simulink model "fft_wideband_real"  (R2012b)
settings: Solver=ode45  StartTime=0.0  StopTime=19999  RelTol=1e-3
undefined symbols (not defined in the file): fft_wideband_real_shift_schedule_user_data_out
libraries: xbsIndex_r4 x8703, xbsReplacements_r4 x36, xps_library x24, dspsigops x16, simulink_xsg_bridge x1
(part 1 of 51)
settings Model: Creator=sgowda  LastModifiedBy=sgowda

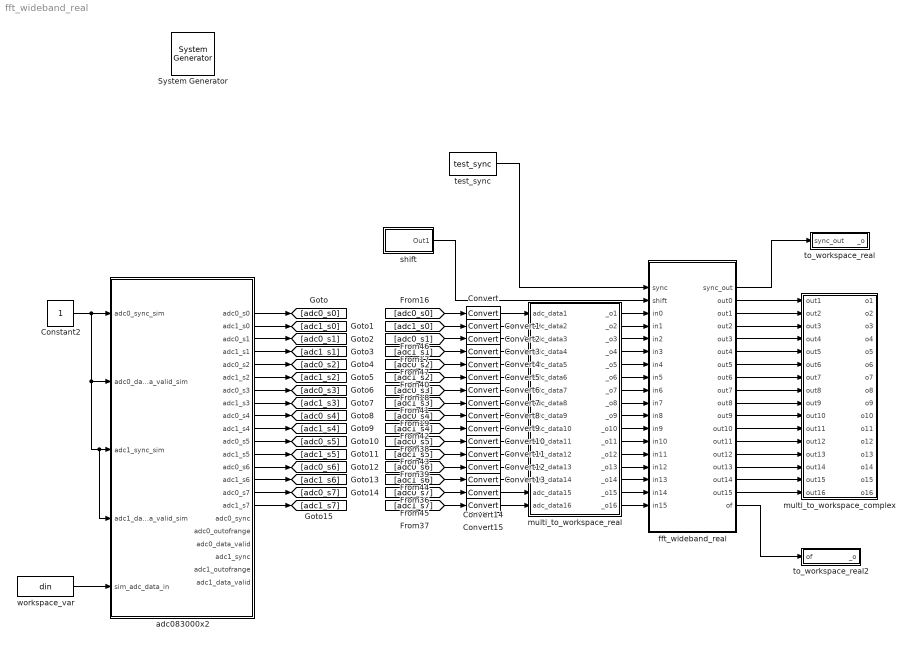
== system fft_wideband_real ==
  " System Generator" : xbsIndex_r4/ System Generator  Tag=genX  xilinxfamily=Kintex7  part=xc7k325t  speed=-3  package=fbg676  synthesis_tool=XST  clock_wrapper=Clock Enables  directory=./netlist  proj_type=Project Navigator  Synth_file=XST Defaults  Impl_file=ISE Defaults  testbench=off  simulink_period=1  sysclk_period=10  dcm_input_clock_period=10  incr_netlist=off  trim_vbits=Everywhere in SubSystem  dbl_ovrd=According to Block Masks  core_generation=According to Block Masks  run_coregen=off  deprecated_control=off  eval_field=0  block_type=sysgen
  Constant2 : Constant
  Convert{,1..15} (16 alike) : xbsIndex_r4/Convert  gui_display_data_type=Fixed-point  arith_type="Signed  (2's comp)"  n_bits=18  bin_pt=17  float_type=Single  exp_bits=8  fraction_bits=24  quantization=Truncate  overflow=Wrap  en=off  latency=0  dbl_ovrd=off  pipeline=off  block_type=convert
  adc083000x2 : Subsystem  Tag=xps:adc083000x2  mask(adc_083000x2){use_adc0=on, use_adc1=on, demux_adc=off, clock_sync=on, verbose=off, using_ctrl=off, adc_clk_rate=1500, sample_period=1, bit_width=8}
      mask prompts: use_adc0 "Use ZD0K0?"; use_adc1 "Use ZDOK1?"; demux_adc "Demux ADCs by 2?"; clock_sync "Interleave 2 ADC boards?"; verbose "Verbose Block Creation?"; using_ctrl "Add ports for control registers?"; adc_clk_rate "ADC clock rate (MHz)"; sample_period "Sample Period"; bit_width "Output Bit Width"
      mask help:
      | The ADC block converts analog inputs to digital outputs.
      | Every clock cycle, the inputs are sampled and digitized to
      | 8 bit binary point numbers in the range of [-1, 1).
      |
      | Online block-specific documentation: http://casper.berkeley.edu/wiki/Adc083000
      mask init:
      | adc083000_mask;
      mask Help: eval('xlWeb([getenv(''MLIB_ROOT''), ''\doc\html\sys_adc\sys_adc.html''])')
  fft_wideband_real : Subsystem
  multi_to_workspace_complex : Subsystem  mask{var_name=out, n_bits=18, bin_pt=17, n_inputs=16}
      mask prompts: var_name "Workspace variable name"; n_bits "# of bits"; bin_pt "Binary Point"; n_inputs "# of inputs"
      mask init:
      | config.source = str2func('multi_mat_output_data_cplx_init_xblock');
      | config.toplevel = gcb();
      | xBlock(config, {config.toplevel, 'var_name', var_name, ...
      |     'n_bits', n_bits, 'bin_pt', bin_pt, 'n_inputs', n_inputs});
  multi_to_workspace_real : Subsystem  mask{var_name=adc_data, n_inputs=16}
      mask prompts: var_name "Workspace variable name"; n_inputs "# of inputs"
      mask init:
      | config.source = str2func('multi_mat_output_data_init_xblock');
      | config.toplevel = gcb();
      | xBlock(config, {config.toplevel, 'var_name', var_name, 'n_inputs', n_inputs});
  shift : Subsystem  mask{shift_schedule=0}
      mask prompts: shift_schedule "Shift schedule"
  test_sync : simulink_xsg_bridge/test_sync
  to_workspace_real : Subsystem  mask{var_name=sync_out}
      mask prompts: var_name "Workspace variable name"
      mask init:
      | config.source = str2func('mat_output_data_init_xblock');
      | config.toplevel = gcb();
      | xBlock(config, {config.toplevel, 'var_name', var_name});
  to_workspace_real2 : Subsystem  mask{var_name=of}
      mask prompts: var_name "Workspace variable name"
      mask init:
      | config.source = str2func('mat_output_data_init_xblock');
      | config.toplevel = gcb();
      | xBlock(config, {config.toplevel, 'var_name', var_name});
  workspace_var : FromWorkspace  VariableName=din
  wires:
  adc083000x2/1(adc0_s0) -> [adc0_s0]
  adc083000x2/2(adc1_s0) -> [adc1_s0]
  adc083000x2/3(adc0_s1) -> [adc0_s1]
  adc083000x2/4(adc1_s1) -> [adc1_s1]
  adc083000x2/5(adc0_s2) -> [adc0_s2]
  adc083000x2/6(adc1_s2) -> [adc1_s2]
  adc083000x2/7(adc0_s3) -> [adc0_s3]
  adc083000x2/8(adc1_s3) -> [adc1_s3]
  adc083000x2/9(adc0_s4) -> [adc0_s4]
  adc083000x2/10(adc1_s4) -> [adc1_s4]
  adc083000x2/11(adc0_s5) -> [adc0_s5]
  adc083000x2/12(adc1_s5) -> [adc1_s5]
  adc083000x2/13(adc0_s6) -> [adc0_s6]
  adc083000x2/14(adc1_s6) -> [adc1_s6]
  adc083000x2/15(adc0_s7) -> [adc0_s7]
  adc083000x2/16(adc1_s7) -> [adc1_s7]
  Constant2/1 -> adc083000x2/2(adc0_data_valid_sim), adc083000x2/3(adc1_sync_sim), adc083000x2/4(adc1_data_valid_sim), adc083000x2/1(adc0_sync_sim)
  workspace_var/1 -> adc083000x2/5(sim_adc_data_in)
  [adc0_s0] -> Convert/1
  [adc1_s0] -> Convert1/1
  [adc0_s1] -> Convert2/1
  [adc1_s1] -> Convert3/1
  [adc0_s2] -> Convert4/1
  [adc1_s2] -> Convert5/1
  [adc0_s3] -> Convert6/1
  [adc1_s3] -> Convert7/1
  [adc0_s4] -> Convert8/1
  [adc1_s4] -> Convert9/1
  [adc0_s5] -> Convert10/1
  [adc1_s5] -> Convert11/1
  [adc0_s6] -> Convert12/1
  [adc1_s6] -> Convert13/1
  [adc0_s7] -> Convert14/1
  [adc1_s7] -> Convert15/1
  test_sync/1 -> fft_wideband_real/1(sync)
  fft_wideband_real/1(sync_out) -> to_workspace_real/1(sync_out)
  shift/1(Out1) -> fft_wideband_real/2(shift)
  fft_wideband_real/2(out0) -> multi_to_workspace_complex/1(out1)
  fft_wideband_real/3(out1) -> multi_to_workspace_complex/2(out2)
  fft_wideband_real/4(out2) -> multi_to_workspace_complex/3(out3)
  fft_wideband_real/5(out3) -> multi_to_workspace_complex/4(out4)
  fft_wideband_real/6(out4) -> multi_to_workspace_complex/5(out5)
  fft_wideband_real/7(out5) -> multi_to_workspace_complex/6(out6)
  fft_wideband_real/8(out6) -> multi_to_workspace_complex/7(out7)
  fft_wideband_real/9(out7) -> multi_to_workspace_complex/8(out8)
  fft_wideband_real/10(out8) -> multi_to_workspace_complex/9(out9)
  fft_wideband_real/11(out9) -> multi_to_workspace_complex/10(out10)
  fft_wideband_real/12(out10) -> multi_to_workspace_complex/11(out11)
  fft_wideband_real/13(out11) -> multi_to_workspace_complex/12(out12)
  fft_wideband_real/14(out12) -> multi_to_workspace_complex/13(out13)
  fft_wideband_real/15(out13) -> multi_to_workspace_complex/14(out14)
  fft_wideband_real/16(out14) -> multi_to_workspace_complex/15(out15)
  fft_wideband_real/17(out15) -> multi_to_workspace_complex/16(out16)
  fft_wideband_real/18(of) -> to_workspace_real2/1(of)
  Convert3/1 -> multi_to_workspace_real/4(adc_data4)
  Convert9/1 -> multi_to_workspace_real/10(adc_data10)
  Convert13/1 -> multi_to_workspace_real/14(adc_data14)
  Convert14/1 -> multi_to_workspace_real/15(adc_data15)
  Convert15/1 -> multi_to_workspace_real/16(adc_data16)
  Convert5/1 -> multi_to_workspace_real/6(adc_data6)
  Convert1/1 -> multi_to_workspace_real/2(adc_data2)
  Convert11/1 -> multi_to_workspace_real/12(adc_data12)
  Convert/1 -> multi_to_workspace_real/1(adc_data1)
  Convert10/1 -> multi_to_workspace_real/11(adc_data11)
  Convert12/1 -> multi_to_workspace_real/13(adc_data13)
  Convert2/1 -> multi_to_workspace_real/3(adc_data3)
  Convert4/1 -> multi_to_workspace_real/5(adc_data5)
  Convert6/1 -> multi_to_workspace_real/7(adc_data7)
  Convert7/1 -> multi_to_workspace_real/8(adc_data8)
  Convert8/1 -> multi_to_workspace_real/9(adc_data9)
  multi_to_workspace_real/13(_o13) -> fft_wideband_real/15(in12)
  multi_to_workspace_real/11(_o11) -> fft_wideband_real/13(in10)
  multi_to_workspace_real/3(_o3) -> fft_wideband_real/5(in2)
  multi_to_workspace_real/1(_o1) -> fft_wideband_real/3(in0)
  multi_to_workspace_real/4(_o4) -> fft_wideband_real/6(in3)
  multi_to_workspace_real/5(_o5) -> fft_wideband_real/7(in4)
  multi_to_workspace_real/8(_o8) -> fft_wideband_real/10(in7)
  multi_to_workspace_real/7(_o7) -> fft_wideband_real/9(in6)
  multi_to_workspace_real/14(_o14) -> fft_wideband_real/16(in13)
  multi_to_workspace_real/12(_o12) -> fft_wideband_real/14(in11)
  multi_to_workspace_real/16(_o16) -> fft_wideband_real/18(in15)
  multi_to_workspace_real/15(_o15) -> fft_wideband_real/17(in14)
  multi_to_workspace_real/6(_o6) -> fft_wideband_real/8(in5)
  multi_to_workspace_real/9(_o9) -> fft_wideband_real/11(in8)
  multi_to_workspace_real/2(_o2) -> fft_wideband_real/4(in1)
  multi_to_workspace_real/10(_o10) -> fft_wideband_real/12(in9)

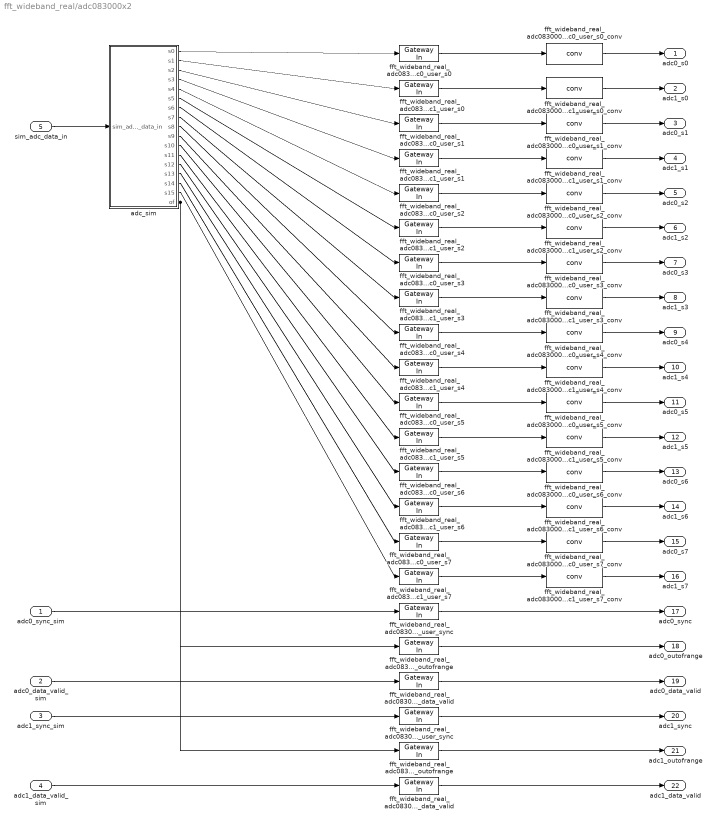
== system fft_wideband_real/adc083000x2 ==
  adc0_sync_sim : Inport
  adc0_data_valid_sim : Inport  Port=2
  adc1_sync_sim : Inport  Port=3
  adc1_data_valid_sim : Inport  Port=4
  sim_adc_data_in : Inport  Port=5
  adc_sim : Subsystem  AncestorBlock=xps_library/ADCs/adc_sim  mask(adc_sim){nStreams=16, bit_width=8}
      mask prompts: nStreams "Number of Output Streams"; bit_width "Sample Bit Width"
      mask help:
      | This block simulates the behavior of a demuxed ADC, which takes
      | as input a waveform and returns digital samples in parallel at
      | a slower rate.
      |
      | This block is used to simulate the behavior
      mask init:
      | adc_sim_init(gcb, ...
      |     'nStreams', nStreams, ...
      |     'bit_width', bit_width);
  fft_wideband_real_adc083000x2_adc0_user_data_valid : xbsIndex_r4/Gateway In  gui_display_data_type=Fixed-point  arith_type=Unsigned  n_bits=1  bin_pt=0  preci_type=Single  exp_width=8  frac_width=24  quantization="Round  (unbiased: +/- Inf)"  overflow=Saturate  period=1  dbl_ovrd=off  timing_constraint=None  locs_specified=off  LOCs={}  UseAsADC=off  ADCChannel='1'  inherit_from_input=off  hdl_port=on  block_type=gatewayin
  fft_wideband_real_adc083000x2_adc0_user_outofrange : xbsIndex_r4/Gateway In  gui_display_data_type=Fixed-point  arith_type=Unsigned  n_bits=4  bin_pt=0  preci_type=Single  exp_width=8  frac_width=24  quantization="Round  (unbiased: +/- Inf)"  overflow=Saturate  period=1  dbl_ovrd=off  timing_constraint=None  locs_specified=off  LOCs={}  UseAsADC=off  ADCChannel='1'  inherit_from_input=off  hdl_port=on  block_type=gatewayin
  fft_wideband_real_adc083000x2_adc0_user_s{0..7} (8 alike) : xbsIndex_r4/Gateway In  gui_display_data_type=Fixed-point  arith_type=Unsigned  n_bits=8  bin_pt=0  preci_type=Single  exp_width=8  frac_width=24  quantization="Round  (unbiased: +/- Inf)"  overflow=Saturate  period=1  dbl_ovrd=off  timing_constraint=None  locs_specified=off  LOCs={}  UseAsADC=off  ADCChannel='1'  inherit_from_input=off  hdl_port=on  block_type=gatewayin
  fft_wideband_real_adc083000x2_adc0_user_s0_conv : xps_library/ADCs/conv  bit_width=8
  fft_wideband_real_adc083000x2_adc0_user_s1_conv : xps_library/ADCs/conv  bit_width=8
  fft_wideband_real_adc083000x2_adc0_user_s2_conv : xps_library/ADCs/conv  bit_width=8
  fft_wideband_real_adc083000x2_adc0_user_s3_conv : xps_library/ADCs/conv  bit_width=8
  fft_wideband_real_adc083000x2_adc0_user_s4_conv : xps_library/ADCs/conv  bit_width=8
  fft_wideband_real_adc083000x2_adc0_user_s5_conv : xps_library/ADCs/conv  bit_width=8
  fft_wideband_real_adc083000x2_adc0_user_s6_conv : xps_library/ADCs/conv  bit_width=8
  fft_wideband_real_adc083000x2_adc0_user_s7_conv : xps_library/ADCs/conv  bit_width=8
  fft_wideband_real_adc083000x2_adc0_user_sync : xbsIndex_r4/Gateway In  gui_display_data_type=Fixed-point  arith_type=Unsigned  n_bits=4  bin_pt=0  preci_type=Single  exp_width=8  frac_width=24  quantization="Round  (unbiased: +/- Inf)"  overflow=Saturate  period=1  dbl_ovrd=off  timing_constraint=None  locs_specified=off  LOCs={}  UseAsADC=off  ADCChannel='1'  inherit_from_input=off  hdl_port=on  block_type=gatewayin
  fft_wideband_real_adc083000x2_adc1_user_data_valid : xbsIndex_r4/Gateway In  gui_display_data_type=Fixed-point  arith_type=Unsigned  n_bits=1  bin_pt=0  preci_type=Single  exp_width=8  frac_width=24  quantization="Round  (unbiased: +/- Inf)"  overflow=Saturate  period=1  dbl_ovrd=off  timing_constraint=None  locs_specified=off  LOCs={}  UseAsADC=off  ADCChannel='1'  inherit_from_input=off  hdl_port=on  block_type=gatewayin
  fft_wideband_real_adc083000x2_adc1_user_outofrange : xbsIndex_r4/Gateway In  gui_display_data_type=Fixed-point  arith_type=Unsigned  n_bits=4  bin_pt=0  preci_type=Single  exp_width=8  frac_width=24  quantization="Round  (unbiased: +/- Inf)"  overflow=Saturate  period=1  dbl_ovrd=off  timing_constraint=None  locs_specified=off  LOCs={}  UseAsADC=off  ADCChannel='1'  inherit_from_input=off  hdl_port=on  block_type=gatewayin
  fft_wideband_real_adc083000x2_adc1_user_s{0..7} (8 alike) : xbsIndex_r4/Gateway In  gui_display_data_type=Fixed-point  arith_type=Unsigned  n_bits=8  bin_pt=0  preci_type=Single  exp_width=8  frac_width=24  quantization="Round  (unbiased: +/- Inf)"  overflow=Saturate  period=1  dbl_ovrd=off  timing_constraint=None  locs_specified=off  LOCs={}  UseAsADC=off  ADCChannel='1'  inherit_from_input=off  hdl_port=on  block_type=gatewayin
  fft_wideband_real_adc083000x2_adc1_user_s0_conv : xps_library/ADCs/conv  bit_width=8
  fft_wideband_real_adc083000x2_adc1_user_s1_conv : xps_library/ADCs/conv  bit_width=8
  fft_wideband_real_adc083000x2_adc1_user_s2_conv : xps_library/ADCs/conv  bit_width=8
  fft_wideband_real_adc083000x2_adc1_user_s3_conv : xps_library/ADCs/conv  bit_width=8
  fft_wideband_real_adc083000x2_adc1_user_s4_conv : xps_library/ADCs/conv  bit_width=8
  fft_wideband_real_adc083000x2_adc1_user_s5_conv : xps_library/ADCs/conv  bit_width=8
  fft_wideband_real_adc083000x2_adc1_user_s6_conv : xps_library/ADCs/conv  bit_width=8
  fft_wideband_real_adc083000x2_adc1_user_s7_conv : xps_library/ADCs/conv  bit_width=8
  fft_wideband_real_adc083000x2_adc1_user_sync : xbsIndex_r4/Gateway In  gui_display_data_type=Fixed-point  arith_type=Unsigned  n_bits=4  bin_pt=0  preci_type=Single  exp_width=8  frac_width=24  quantization="Round  (unbiased: +/- Inf)"  overflow=Saturate  period=1  dbl_ovrd=off  timing_constraint=None  locs_specified=off  LOCs={}  UseAsADC=off  ADCChannel='1'  inherit_from_input=off  hdl_port=on  block_type=gatewayin
  adc0_s0 : Outport
  adc1_s0 : Outport  Port=2
  adc0_s1 : Outport  Port=3
  adc1_s1 : Outport  Port=4
  adc0_s2 : Outport  Port=5
  adc1_s2 : Outport  Port=6
  adc0_s3 : Outport  Port=7
  adc1_s3 : Outport  Port=8
  adc0_s4 : Outport  Port=9
  adc1_s4 : Outport  Port=10
  adc0_s5 : Outport  Port=11
  adc1_s5 : Outport  Port=12
  adc0_s6 : Outport  Port=13
  adc1_s6 : Outport  Port=14
  adc0_s7 : Outport  Port=15
  adc1_s7 : Outport  Port=16
  adc0_sync : Outport  Port=17
  adc0_outofrange : Outport  Port=18
  adc0_data_valid : Outport  Port=19
  adc1_sync : Outport  Port=20
  adc1_outofrange : Outport  Port=21
  adc1_data_valid : Outport  Port=22
  wires:
  sim_adc_data_in/1 -> adc_sim/1(sim_adc_data_in)
  adc_sim/1(s0) -> fft_wideband_real_adc083000x2_adc0_user_s0/1
  fft_wideband_real_adc083000x2_adc0_user_s0/1 -> fft_wideband_real_adc083000x2_adc0_user_s0_conv/1
  fft_wideband_real_adc083000x2_adc0_user_s0_conv/1 -> adc0_s0/1
  adc_sim/2(s1) -> fft_wideband_real_adc083000x2_adc1_user_s0/1
  fft_wideband_real_adc083000x2_adc1_user_s0/1 -> fft_wideband_real_adc083000x2_adc1_user_s0_conv/1
  fft_wideband_real_adc083000x2_adc1_user_s0_conv/1 -> adc1_s0/1
  adc_sim/3(s2) -> fft_wideband_real_adc083000x2_adc0_user_s1/1
  fft_wideband_real_adc083000x2_adc0_user_s1/1 -> fft_wideband_real_adc083000x2_adc0_user_s1_conv/1
  fft_wideband_real_adc083000x2_adc0_user_s1_conv/1 -> adc0_s1/1
  adc_sim/4(s3) -> fft_wideband_real_adc083000x2_adc1_user_s1/1
  fft_wideband_real_adc083000x2_adc1_user_s1/1 -> fft_wideband_real_adc083000x2_adc1_user_s1_conv/1
  fft_wideband_real_adc083000x2_adc1_user_s1_conv/1 -> adc1_s1/1
  adc_sim/5(s4) -> fft_wideband_real_adc083000x2_adc0_user_s2/1
  fft_wideband_real_adc083000x2_adc0_user_s2/1 -> fft_wideband_real_adc083000x2_adc0_user_s2_conv/1
  fft_wideband_real_adc083000x2_adc0_user_s2_conv/1 -> adc0_s2/1
  adc_sim/6(s5) -> fft_wideband_real_adc083000x2_adc1_user_s2/1
  fft_wideband_real_adc083000x2_adc1_user_s2/1 -> fft_wideband_real_adc083000x2_adc1_user_s2_conv/1
  fft_wideband_real_adc083000x2_adc1_user_s2_conv/1 -> adc1_s2/1
  adc_sim/7(s6) -> fft_wideband_real_adc083000x2_adc0_user_s3/1
  fft_wideband_real_adc083000x2_adc0_user_s3/1 -> fft_wideband_real_adc083000x2_adc0_user_s3_conv/1
  fft_wideband_real_adc083000x2_adc0_user_s3_conv/1 -> adc0_s3/1
  adc_sim/8(s7) -> fft_wideband_real_adc083000x2_adc1_user_s3/1
  fft_wideband_real_adc083000x2_adc1_user_s3/1 -> fft_wideband_real_adc083000x2_adc1_user_s3_conv/1
  fft_wideband_real_adc083000x2_adc1_user_s3_conv/1 -> adc1_s3/1
  adc_sim/9(s8) -> fft_wideband_real_adc083000x2_adc0_user_s4/1
  fft_wideband_real_adc083000x2_adc0_user_s4/1 -> fft_wideband_real_adc083000x2_adc0_user_s4_conv/1
  fft_wideband_real_adc083000x2_adc0_user_s4_conv/1 -> adc0_s4/1
  adc_sim/10(s9) -> fft_wideband_real_adc083000x2_adc1_user_s4/1
  fft_wideband_real_adc083000x2_adc1_user_s4/1 -> fft_wideband_real_adc083000x2_adc1_user_s4_conv/1
  fft_wideband_real_adc083000x2_adc1_user_s4_conv/1 -> adc1_s4/1
  adc_sim/11(s10) -> fft_wideband_real_adc083000x2_adc0_user_s5/1
  fft_wideband_real_adc083000x2_adc0_user_s5/1 -> fft_wideband_real_adc083000x2_adc0_user_s5_conv/1
  fft_wideband_real_adc083000x2_adc0_user_s5_conv/1 -> adc0_s5/1
  adc_sim/12(s11) -> fft_wideband_real_adc083000x2_adc1_user_s5/1
  fft_wideband_real_adc083000x2_adc1_user_s5/1 -> fft_wideband_real_adc083000x2_adc1_user_s5_conv/1
  fft_wideband_real_adc083000x2_adc1_user_s5_conv/1 -> adc1_s5/1
  adc_sim/13(s12) -> fft_wideband_real_adc083000x2_adc0_user_s6/1
  fft_wideband_real_adc083000x2_adc0_user_s6/1 -> fft_wideband_real_adc083000x2_adc0_user_s6_conv/1
  fft_wideband_real_adc083000x2_adc0_user_s6_conv/1 -> adc0_s6/1
  adc_sim/14(s13) -> fft_wideband_real_adc083000x2_adc1_user_s6/1
  fft_wideband_real_adc083000x2_adc1_user_s6/1 -> fft_wideband_real_adc083000x2_adc1_user_s6_conv/1
  fft_wideband_real_adc083000x2_adc1_user_s6_conv/1 -> adc1_s6/1
  adc_sim/15(s14) -> fft_wideband_real_adc083000x2_adc0_user_s7/1
  fft_wideband_real_adc083000x2_adc0_user_s7/1 -> fft_wideband_real_adc083000x2_adc0_user_s7_conv/1
  fft_wideband_real_adc083000x2_adc0_user_s7_conv/1 -> adc0_s7/1
  adc_sim/16(s15) -> fft_wideband_real_adc083000x2_adc1_user_s7/1
  fft_wideband_real_adc083000x2_adc1_user_s7/1 -> fft_wideband_real_adc083000x2_adc1_user_s7_conv/1
  fft_wideband_real_adc083000x2_adc1_user_s7_conv/1 -> adc1_s7/1
  adc0_sync_sim/1 -> fft_wideband_real_adc083000x2_adc0_user_sync/1
  fft_wideband_real_adc083000x2_adc0_user_sync/1 -> adc0_sync/1
  adc_sim/17(of) -> fft_wideband_real_adc083000x2_adc0_user_outofrange/1, fft_wideband_real_adc083000x2_adc1_user_outofrange/1
  fft_wideband_real_adc083000x2_adc0_user_outofrange/1 -> adc0_outofrange/1
  adc0_data_valid_sim/1 -> fft_wideband_real_adc083000x2_adc0_user_data_valid/1
  fft_wideband_real_adc083000x2_adc0_user_data_valid/1 -> adc0_data_valid/1
  adc1_sync_sim/1 -> fft_wideband_real_adc083000x2_adc1_user_sync/1
  fft_wideband_real_adc083000x2_adc1_user_sync/1 -> adc1_sync/1
  fft_wideband_real_adc083000x2_adc1_user_outofrange/1 -> adc1_outofrange/1
  adc1_data_valid_sim/1 -> fft_wideband_real_adc083000x2_adc1_user_data_valid/1
  fft_wideband_real_adc083000x2_adc1_user_data_valid/1 -> adc1_data_valid/1

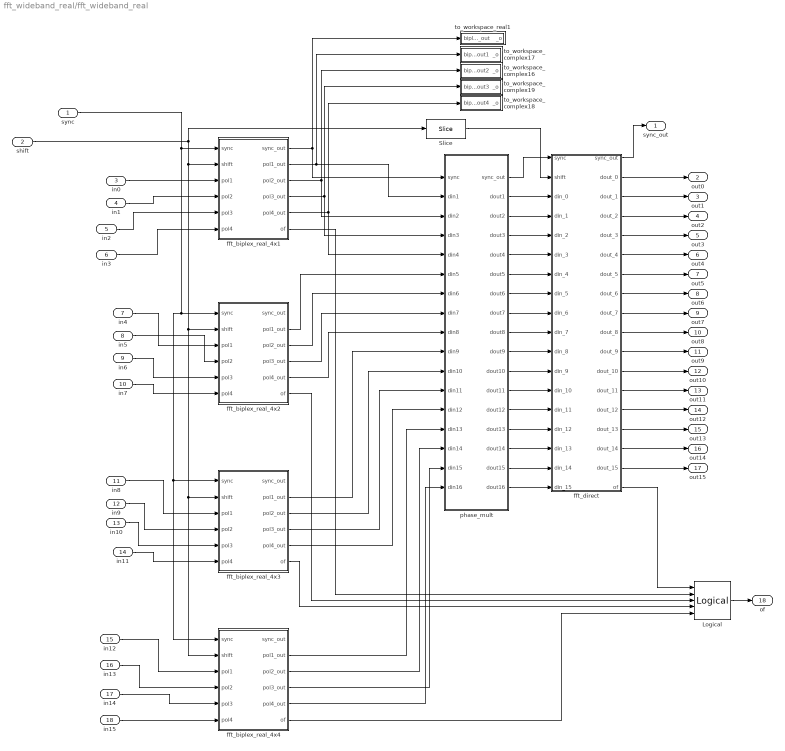
== system fft_wideband_real/fft_wideband_real ==
  sync : Inport
  shift : Inport  Port=2
  in0 : Inport  Port=3
  in1 : Inport  Port=4
  in2 : Inport  Port=5
  in3 : Inport  Port=6
  in4 : Inport  Port=7
  in5 : Inport  Port=8
  in6 : Inport  Port=9
  in7 : Inport  Port=10
  in8 : Inport  Port=11
  in9 : Inport  Port=12
  in10 : Inport  Port=13
  in11 : Inport  Port=14
  in12 : Inport  Port=15
  in13 : Inport  Port=16
  in14 : Inport  Port=17
  in15 : Inport  Port=18
  Logical : xbsIndex_r4/Logical  logical_function=OR  inputs=5  en=off  latency=0  precision=Full  arith_type=Unsigned  n_bits=16  bin_pt=0  align_bp=on  dbl_ovrd=off  block_type=logical
  Slice : xbsIndex_r4/Slice  nbits=4  boolean_output=off  mode=Lower Bit Location + Width  bit1=0  base1=MSB of Input  bit0=6  base0=LSB of Input  dbl_ovrd=off  block_type=slice
  fft_biplex_real_4x1 : Subsystem
      settings: AttributesFormatString=|
      | Virtex5
      | 6 stages
      | [18,18]
      | Round  (unbiased: +/- Inf)
      | Saturate
      | 0 0 0 0 0 0 0 0
  fft_biplex_real_4x2 : Subsystem
      settings: AttributesFormatString=|
      | Virtex5
      | 6 stages
      | [18,18]
      | Round  (unbiased: +/- Inf)
      | Saturate
      | 0 0 0 0 0 0 0 0
  fft_biplex_real_4x3 : Subsystem
      settings: AttributesFormatString=|
      | Virtex5
      | 6 stages
      | [18,18]
      | Round  (unbiased: +/- Inf)
      | Saturate
      | 0 0 0 0 0 0 0 0
  fft_biplex_real_4x4 : Subsystem
      settings: AttributesFormatString=|
      | Virtex5
      | 6 stages
      | [18,18]
      | Round  (unbiased: +/- Inf)
      | Saturate
      | 0 0 0 0 0 0 0 0
  fft_direct : Subsystem
  phase_mult : Subsystem
  to_workspace_complex16 : Subsystem  mask{var_name=biplex_out2, n_bits=18, bin_pt=17}
      mask prompts: var_name "Workspace variable name"; n_bits "# of bits"; bin_pt "Binary Point"
      mask init:
      | config.source = str2func('mat_output_data_cplx_init_xblock');
      | config.toplevel = gcb();
      | xBlock(config, {config.toplevel, 'var_name', var_name, ...
      |     'n_bits', n_bits, 'bin_pt', bin_pt});
  to_workspace_complex17 : Subsystem  mask{var_name=biplex_out1, n_bits=18, bin_pt=17}
      mask prompts: var_name "Workspace variable name"; n_bits "# of bits"; bin_pt "Binary Point"
      mask init:
      | config.source = str2func('mat_output_data_cplx_init_xblock');
      | config.toplevel = gcb();
      | xBlock(config, {config.toplevel, 'var_name', var_name, ...
      |     'n_bits', n_bits, 'bin_pt', bin_pt});
  to_workspace_complex18 : Subsystem  mask{var_name=biplex_out4, n_bits=18, bin_pt=17}
      mask prompts: var_name "Workspace variable name"; n_bits "# of bits"; bin_pt "Binary Point"
      mask init:
      | config.source = str2func('mat_output_data_cplx_init_xblock');
      | config.toplevel = gcb();
      | xBlock(config, {config.toplevel, 'var_name', var_name, ...
      |     'n_bits', n_bits, 'bin_pt', bin_pt});
  to_workspace_complex19 : Subsystem  mask{var_name=biplex_out3, n_bits=18, bin_pt=17}
      mask prompts: var_name "Workspace variable name"; n_bits "# of bits"; bin_pt "Binary Point"
      mask init:
      | config.source = str2func('mat_output_data_cplx_init_xblock');
      | config.toplevel = gcb();
      | xBlock(config, {config.toplevel, 'var_name', var_name, ...
      |     'n_bits', n_bits, 'bin_pt', bin_pt});
  to_workspace_real1 : Subsystem  mask{var_name=biplex_sync_out}
      mask prompts: var_name "Workspace variable name"
      mask init:
      | config.source = str2func('mat_output_data_init_xblock');
      | config.toplevel = gcb();
      | xBlock(config, {config.toplevel, 'var_name', var_name});
  sync_out : Outport
  out0 : Outport  Port=2
  out1 : Outport  Port=3
  out2 : Outport  Port=4
  out3 : Outport  Port=5
  out4 : Outport  Port=6
  out5 : Outport  Port=7
  out6 : Outport  Port=8
  out7 : Outport  Port=9
  out8 : Outport  Port=10
  out9 : Outport  Port=11
  out10 : Outport  Port=12
  out11 : Outport  Port=13
  out12 : Outport  Port=14
  out13 : Outport  Port=15
  out14 : Outport  Port=16
  out15 : Outport  Port=17
  of : Outport  Port=18
  wires:
  in2/1 -> fft_biplex_real_4x1/5(pol3)
  in0/1 -> fft_biplex_real_4x1/3(pol1)
  in1/1 -> fft_biplex_real_4x1/4(pol2)
  in4/1 -> fft_biplex_real_4x2/3(pol1)
  in6/1 -> fft_biplex_real_4x2/5(pol3)
  in8/1 -> fft_biplex_real_4x3/3(pol1)
  in10/1 -> fft_biplex_real_4x3/5(pol3)
  in11/1 -> fft_biplex_real_4x3/6(pol4)
  in12/1 -> fft_biplex_real_4x4/3(pol1)
  in13/1 -> fft_biplex_real_4x4/4(pol2)
  in14/1 -> fft_biplex_real_4x4/5(pol3)
  in15/1 -> fft_biplex_real_4x4/6(pol4)
  fft_biplex_real_4x2/2(pol1_out) -> phase_mult/6(din5)
  fft_biplex_real_4x2/3(pol2_out) -> phase_mult/7(din6)
  fft_biplex_real_4x2/4(pol3_out) -> phase_mult/8(din7)
  fft_biplex_real_4x2/5(pol4_out) -> phase_mult/9(din8)
  fft_biplex_real_4x3/2(pol1_out) -> phase_mult/10(din9)
  fft_biplex_real_4x3/3(pol2_out) -> phase_mult/11(din10)
  fft_biplex_real_4x3/4(pol3_out) -> phase_mult/12(din11)
  fft_biplex_real_4x3/5(pol4_out) -> phase_mult/13(din12)
  fft_biplex_real_4x4/2(pol1_out) -> phase_mult/14(din13)
  fft_biplex_real_4x4/3(pol2_out) -> phase_mult/15(din14)
  fft_biplex_real_4x4/4(pol3_out) -> phase_mult/16(din15)
  fft_biplex_real_4x4/5(pol4_out) -> phase_mult/17(din16)
  phase_mult/1(sync_out) -> fft_direct/1(sync)
  shift/1 -> fft_biplex_real_4x1/2(shift), fft_biplex_real_4x2/2(shift), fft_biplex_real_4x4/2(shift), fft_biplex_real_4x3/2(shift), Slice/1
  phase_mult/9(dout8) -> fft_direct/10(din_7)
  phase_mult/10(dout9) -> fft_direct/11(din_8)
  phase_mult/11(dout10) -> fft_direct/12(din_9)
  phase_mult/12(dout11) -> fft_direct/13(din_10)
  phase_mult/13(dout12) -> fft_direct/14(din_11)
  phase_mult/14(dout13) -> fft_direct/15(din_12)
  phase_mult/2(dout1) -> fft_direct/3(din_0)
  phase_mult/3(dout2) -> fft_direct/4(din_1)
  phase_mult/4(dout3) -> fft_direct/5(din_2)
  phase_mult/5(dout4) -> fft_direct/6(din_3)
  phase_mult/6(dout5) -> fft_direct/7(din_4)
  phase_mult/8(dout7) -> fft_direct/9(din_6)
  phase_mult/7(dout6) -> fft_direct/8(din_5)
  phase_mult/16(dout15) -> fft_direct/17(din_14)
  phase_mult/17(dout16) -> fft_direct/18(din_15)
  phase_mult/15(dout14) -> fft_direct/16(din_13)
  sync/1 -> fft_biplex_real_4x1/1(sync), fft_biplex_real_4x2/1(sync), fft_biplex_real_4x4/1(sync), fft_biplex_real_4x3/1(sync)
  fft_direct/1(sync_out) -> sync_out/1
  fft_direct/2(dout_0) -> out0/1
  fft_direct/3(dout_1) -> out1/1
  fft_direct/4(dout_2) -> out2/1
  fft_direct/5(dout_3) -> out3/1
  fft_direct/6(dout_4) -> out4/1
  fft_direct/7(dout_5) -> out5/1
  fft_direct/8(dout_6) -> out6/1
  fft_direct/9(dout_7) -> out7/1
  fft_direct/10(dout_8) -> out8/1
  fft_direct/11(dout_9) -> out9/1
  fft_direct/12(dout_10) -> out10/1
  fft_direct/13(dout_11) -> out11/1
  fft_direct/14(dout_12) -> out12/1
  fft_direct/15(dout_13) -> out13/1
  fft_direct/16(dout_14) -> out14/1
  fft_direct/17(dout_15) -> out15/1
  fft_biplex_real_4x1/2(pol1_out) -> phase_mult/2(din1), to_workspace_complex17/1(biplex_out1)
  fft_biplex_real_4x1/3(pol2_out) -> phase_mult/3(din2), to_workspace_complex16/1(biplex_out2)
  fft_biplex_real_4x1/4(pol3_out) -> phase_mult/4(din3), to_workspace_complex19/1(biplex_out3)
  fft_biplex_real_4x1/5(pol4_out) -> phase_mult/5(din4), to_workspace_complex18/1(biplex_out4)
  fft_biplex_real_4x1/1(sync_out) -> phase_mult/1(sync), to_workspace_real1/1(biplex_sync_out)
  Slice/1 -> fft_direct/2(shift)
  fft_direct/18(of) -> Logical/1
  fft_biplex_real_4x1/6(of) -> Logical/2
  fft_biplex_real_4x2/6(of) -> Logical/3
  fft_biplex_real_4x3/6(of) -> Logical/4
  fft_biplex_real_4x4/6(of) -> Logical/5
  in7/1 -> fft_biplex_real_4x2/6(pol4)
  in5/1 -> fft_biplex_real_4x2/4(pol2)
  in3/1 -> fft_biplex_real_4x1/6(pol4)
  in9/1 -> fft_biplex_real_4x3/4(pol2)
  Logical/1 -> of/1

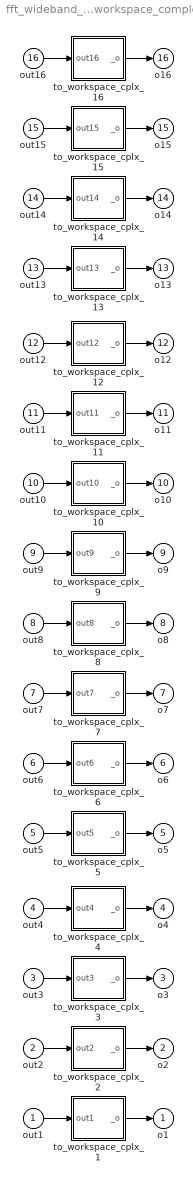
== system fft_wideband_real/multi_to_workspace_complex ==
  out1 : Inport
  out2 : Inport  Port=2
  out3 : Inport  Port=3
  out4 : Inport  Port=4
  out5 : Inport  Port=5
  out6 : Inport  Port=6
  out7 : Inport  Port=7
  out8 : Inport  Port=8
  out9 : Inport  Port=9
  out10 : Inport  Port=10
  out11 : Inport  Port=11
  out12 : Inport  Port=12
  out13 : Inport  Port=13
  out14 : Inport  Port=14
  out15 : Inport  Port=15
  out16 : Inport  Port=16
  to_workspace_cplx_1 : Subsystem
  to_workspace_cplx_10 : Subsystem
  to_workspace_cplx_11 : Subsystem
  to_workspace_cplx_12 : Subsystem
  to_workspace_cplx_13 : Subsystem
  to_workspace_cplx_14 : Subsystem
  to_workspace_cplx_15 : Subsystem
  to_workspace_cplx_16 : Subsystem
  to_workspace_cplx_2 : Subsystem
  to_workspace_cplx_3 : Subsystem
  to_workspace_cplx_4 : Subsystem
  to_workspace_cplx_5 : Subsystem
  to_workspace_cplx_6 : Subsystem
  to_workspace_cplx_7 : Subsystem
  to_workspace_cplx_8 : Subsystem
  to_workspace_cplx_9 : Subsystem
  o1 : Outport
  o2 : Outport  Port=2
  o3 : Outport  Port=3
  o4 : Outport  Port=4
  o5 : Outport  Port=5
  o6 : Outport  Port=6
  o7 : Outport  Port=7
  o8 : Outport  Port=8
  o9 : Outport  Port=9
  o10 : Outport  Port=10
  o11 : Outport  Port=11
  o12 : Outport  Port=12
  o13 : Outport  Port=13
  o14 : Outport  Port=14
  o15 : Outport  Port=15
  o16 : Outport  Port=16
  wires:
  to_workspace_cplx_16/1(_o) -> o16/1
  out16/1 -> to_workspace_cplx_16/1(out16)
  to_workspace_cplx_15/1(_o) -> o15/1
  out15/1 -> to_workspace_cplx_15/1(out15)
  to_workspace_cplx_14/1(_o) -> o14/1
  out14/1 -> to_workspace_cplx_14/1(out14)
  to_workspace_cplx_13/1(_o) -> o13/1
  out13/1 -> to_workspace_cplx_13/1(out13)
  to_workspace_cplx_12/1(_o) -> o12/1
  out12/1 -> to_workspace_cplx_12/1(out12)
  to_workspace_cplx_11/1(_o) -> o11/1
  out11/1 -> to_workspace_cplx_11/1(out11)
  to_workspace_cplx_10/1(_o) -> o10/1
  out10/1 -> to_workspace_cplx_10/1(out10)
  to_workspace_cplx_9/1(_o) -> o9/1
  out9/1 -> to_workspace_cplx_9/1(out9)
  to_workspace_cplx_8/1(_o) -> o8/1
  out8/1 -> to_workspace_cplx_8/1(out8)
  to_workspace_cplx_7/1(_o) -> o7/1
  out7/1 -> to_workspace_cplx_7/1(out7)
  to_workspace_cplx_6/1(_o) -> o6/1
  out6/1 -> to_workspace_cplx_6/1(out6)
  to_workspace_cplx_5/1(_o) -> o5/1
  out5/1 -> to_workspace_cplx_5/1(out5)
  to_workspace_cplx_4/1(_o) -> o4/1
  out4/1 -> to_workspace_cplx_4/1(out4)
  to_workspace_cplx_3/1(_o) -> o3/1
  out3/1 -> to_workspace_cplx_3/1(out3)
  to_workspace_cplx_2/1(_o) -> o2/1
  out2/1 -> to_workspace_cplx_2/1(out2)
  to_workspace_cplx_1/1(_o) -> o1/1
  out1/1 -> to_workspace_cplx_1/1(out1)

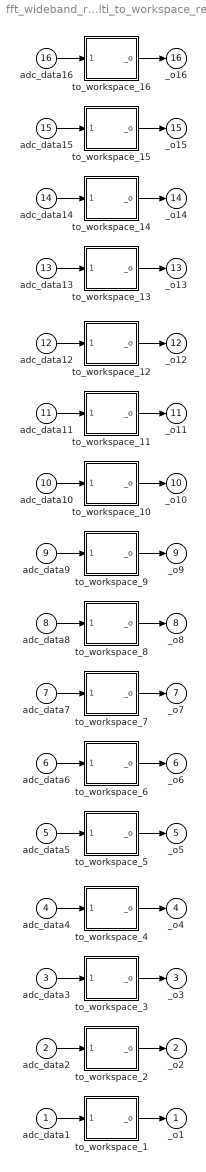
== system fft_wideband_real/multi_to_workspace_real ==
  adc_data1 : Inport
  adc_data2 : Inport  Port=2
  adc_data3 : Inport  Port=3
  adc_data4 : Inport  Port=4
  adc_data5 : Inport  Port=5
  adc_data6 : Inport  Port=6
  adc_data7 : Inport  Port=7
  adc_data8 : Inport  Port=8
  adc_data9 : Inport  Port=9
  adc_data10 : Inport  Port=10
  adc_data11 : Inport  Port=11
  adc_data12 : Inport  Port=12
  adc_data13 : Inport  Port=13
  adc_data14 : Inport  Port=14
  adc_data15 : Inport  Port=15
  adc_data16 : Inport  Port=16
  to_workspace_1 : Subsystem
  to_workspace_10 : Subsystem
  to_workspace_11 : Subsystem
  to_workspace_12 : Subsystem
  to_workspace_13 : Subsystem
  to_workspace_14 : Subsystem
  to_workspace_15 : Subsystem
  to_workspace_16 : Subsystem
  to_workspace_2 : Subsystem
  to_workspace_3 : Subsystem
  to_workspace_4 : Subsystem
  to_workspace_5 : Subsystem
  to_workspace_6 : Subsystem
  to_workspace_7 : Subsystem
  to_workspace_8 : Subsystem
  to_workspace_9 : Subsystem
  _o1 : Outport
  _o2 : Outport  Port=2
  _o3 : Outport  Port=3
  _o4 : Outport  Port=4
  _o5 : Outport  Port=5
  _o6 : Outport  Port=6
  _o7 : Outport  Port=7
  _o8 : Outport  Port=8
  _o9 : Outport  Port=9
  _o10 : Outport  Port=10
  _o11 : Outport  Port=11
  _o12 : Outport  Port=12
  _o13 : Outport  Port=13
  _o14 : Outport  Port=14
  _o15 : Outport  Port=15
  _o16 : Outport  Port=16
  wires:
  to_workspace_16/1(_o) -> _o16/1
  adc_data16/1 -> to_workspace_16/1(adc_data16)
  to_workspace_15/1(_o) -> _o15/1
  adc_data15/1 -> to_workspace_15/1(adc_data15)
  to_workspace_14/1(_o) -> _o14/1
  adc_data14/1 -> to_workspace_14/1(adc_data14)
  to_workspace_13/1(_o) -> _o13/1
  adc_data13/1 -> to_workspace_13/1(adc_data13)
  to_workspace_12/1(_o) -> _o12/1
  adc_data12/1 -> to_workspace_12/1(adc_data12)
  to_workspace_11/1(_o) -> _o11/1
  adc_data11/1 -> to_workspace_11/1(adc_data11)
  to_workspace_10/1(_o) -> _o10/1
  adc_data10/1 -> to_workspace_10/1(adc_data10)
  to_workspace_9/1(_o) -> _o9/1
  adc_data9/1 -> to_workspace_9/1(adc_data9)
  to_workspace_8/1(_o) -> _o8/1
  adc_data8/1 -> to_workspace_8/1(adc_data8)
  to_workspace_7/1(_o) -> _o7/1
  adc_data7/1 -> to_workspace_7/1(adc_data7)
  to_workspace_6/1(_o) -> _o6/1
  adc_data6/1 -> to_workspace_6/1(adc_data6)
  to_workspace_5/1(_o) -> _o5/1
  adc_data5/1 -> to_workspace_5/1(adc_data5)
  to_workspace_4/1(_o) -> _o4/1
  adc_data4/1 -> to_workspace_4/1(adc_data4)
  to_workspace_3/1(_o) -> _o3/1
  adc_data3/1 -> to_workspace_3/1(adc_data3)
  to_workspace_2/1(_o) -> _o2/1
  adc_data2/1 -> to_workspace_2/1(adc_data2)
  to_workspace_1/1(_o) -> _o1/1
  adc_data1/1 -> to_workspace_1/1(adc_data1)

== system fft_wideband_real/shift ==
  Constant : Constant  Value=bin2dec('0110101011')
  schedule : Subsystem  Tag=xps:sw_reg  mask{io_dir=From Processor, arith_type=Unsigned, bitwidth=32, bin_pt=0, sample_period=1, gw_name=fft_wideband_real_shift_schedule_user_data_out}
      mask prompts: io_dir "I/O direction"; arith_type "Data Type"; bitwidth "Data bitwidth"; bin_pt "Data binary point"; sample_period "Sample period"; gw_name "Mask Parameter 6:"
      mask init:
      | register_mask;
      mask TypeOptions io_dir: From Processor | To Processor
      mask TypeOptions arith_type: Unsigned | Signed  (2's comp)
  Out1 : Outport
  wires:
  Constant/1 -> schedule/1(sim_in)
  schedule/1(reg_in) -> Out1/1

== system fft_wideband_real/to_workspace_real ==
  sync_out : Inport
  gateway : xbsIndex_r4/Gateway Out  inherit_from_input=on  hdl_port=off  timing_constraint=None  locs_specified=off  LOCs={}  UseAsDAC=off  DACChannel='1'  block_type=gatewayout
  workspace_input : ToWorkspace  VariableName=sync_out  SampleTime=-1
  _o : Outport
  wires:
  sync_out/1 -> gateway/1, _o/1
  gateway/1 -> workspace_input/1

== system fft_wideband_real/to_workspace_real2 ==
  of : Inport
  gateway : xbsIndex_r4/Gateway Out  inherit_from_input=on  hdl_port=off  timing_constraint=None  locs_specified=off  LOCs={}  UseAsDAC=off  DACChannel='1'  block_type=gatewayout
  workspace_input : ToWorkspace  VariableName=of  SampleTime=-1
  _o : Outport
  wires:
  of/1 -> gateway/1, _o/1
  gateway/1 -> workspace_input/1

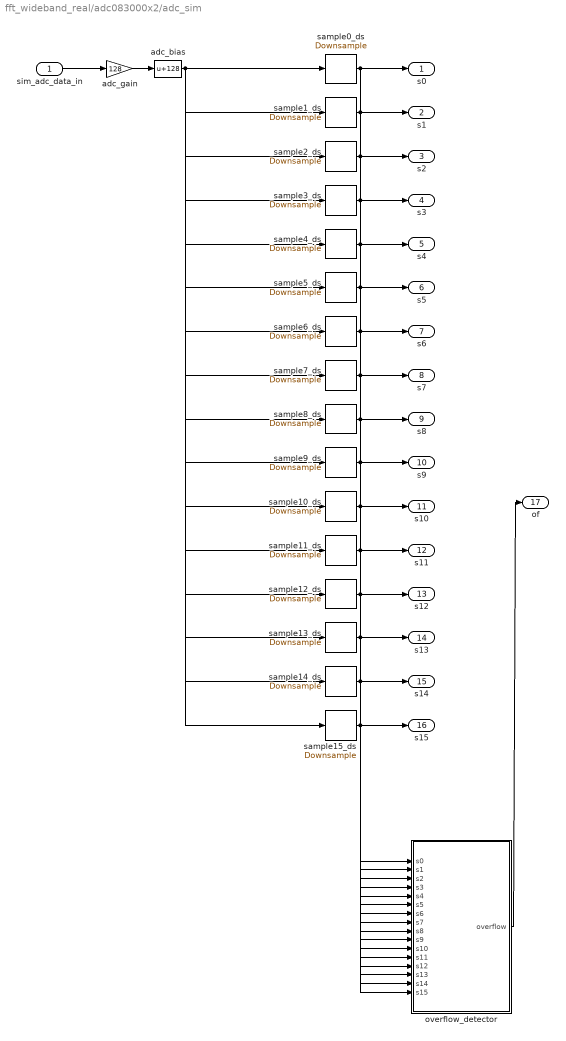
== system fft_wideband_real/adc083000x2/adc_sim ==
  sim_adc_data_in : Inport
  adc_bias : Bias  Bias=128  SaturateOnIntegerOverflow=on
  adc_gain : Gain  Gain=128
  overflow_detector : Subsystem  AncestorBlock=xps_library/ADCs/of_detect_bus  mask(of_detect_bus){nStreams=16, bit_width=8}
      mask prompts: nStreams "Number of Streams"; bit_width "Bit Width"
      mask init:
      | of_detect_bus_init(gcb, ...
      |     'nStreams', nStreams, ...
      |     'bit_width', bit_width);
  sample0_ds : dspsigops/Downsample  N=16  phase=1  RateOptions=Allow multirate processing  smode=Force single rate  fmode=Maintain input frame rate  ic=0
  sample10_ds : dspsigops/Downsample  N=16  phase=11  RateOptions=Allow multirate processing  smode=Force single rate  fmode=Maintain input frame size  ic=0
  sample11_ds : dspsigops/Downsample  N=16  phase=12  RateOptions=Allow multirate processing  smode=Force single rate  fmode=Maintain input frame size  ic=0
  sample12_ds : dspsigops/Downsample  N=16  phase=13  RateOptions=Allow multirate processing  smode=Force single rate  fmode=Maintain input frame size  ic=0
  sample13_ds : dspsigops/Downsample  N=16  phase=14  RateOptions=Allow multirate processing  smode=Force single rate  fmode=Maintain input frame size  ic=0
  sample14_ds : dspsigops/Downsample  N=16  phase=15  RateOptions=Allow multirate processing  smode=Force single rate  fmode=Maintain input frame size  ic=0
  sample15_ds : dspsigops/Downsample  N=16  phase=0  RateOptions=Allow multirate processing  smode=Force single rate  fmode=Maintain input frame size  ic=0
  sample1_ds : dspsigops/Downsample  N=16  phase=2  RateOptions=Allow multirate processing  smode=Force single rate  fmode=Maintain input frame rate  ic=0
  sample2_ds : dspsigops/Downsample  N=16  phase=3  RateOptions=Allow multirate processing  smode=Force single rate  fmode=Maintain input frame rate  ic=0
  sample3_ds : dspsigops/Downsample  N=16  phase=4  RateOptions=Allow multirate processing  smode=Force single rate  fmode=Maintain input frame rate  ic=0
  sample4_ds : dspsigops/Downsample  N=16  phase=5  RateOptions=Allow multirate processing  smode=Force single rate  fmode=Maintain input frame rate  ic=0
  sample5_ds : dspsigops/Downsample  N=16  phase=6  RateOptions=Allow multirate processing  smode=Force single rate  fmode=Maintain input frame rate  ic=0
  sample6_ds : dspsigops/Downsample  N=16  phase=7  RateOptions=Allow multirate processing  smode=Force single rate  fmode=Maintain input frame rate  ic=0
  sample7_ds : dspsigops/Downsample  N=16  phase=8  RateOptions=Allow multirate processing  smode=Force single rate  fmode=Maintain input frame rate  ic=0
  sample8_ds : dspsigops/Downsample  N=16  phase=9  RateOptions=Allow multirate processing  smode=Force single rate  fmode=Maintain input frame size  ic=0
  sample9_ds : dspsigops/Downsample  N=16  phase=10  RateOptions=Allow multirate processing  smode=Force single rate  fmode=Maintain input frame size  ic=0
  s0 : Outport
  s1 : Outport  Port=2
  s2 : Outport  Port=3
  s3 : Outport  Port=4
  s4 : Outport  Port=5
  s5 : Outport  Port=6
  s6 : Outport  Port=7
  s7 : Outport  Port=8
  s8 : Outport  Port=9
  s9 : Outport  Port=10
  s10 : Outport  Port=11
  s11 : Outport  Port=12
  s12 : Outport  Port=13
  s13 : Outport  Port=14
  s14 : Outport  Port=15
  s15 : Outport  Port=16
  of : Outport  Port=17
  wires:
  sim_adc_data_in/1 -> adc_gain/1
  adc_gain/1 -> adc_bias/1
  overflow_detector/1(overflow) -> of/1
  adc_bias/1 -> sample0_ds/1, sample1_ds/1, sample2_ds/1, sample3_ds/1, sample4_ds/1, sample5_ds/1, sample6_ds/1, sample7_ds/1, sample8_ds/1, sample9_ds/1, sample10_ds/1, sample11_ds/1, sample12_ds/1, sample13_ds/1, sample14_ds/1, sample15_ds/1
  sample0_ds/1 -> overflow_detector/1(s0), s0/1
  sample1_ds/1 -> overflow_detector/2(s1), s1/1
  sample2_ds/1 -> overflow_detector/3(s2), s2/1
  sample3_ds/1 -> overflow_detector/4(s3), s3/1
  sample4_ds/1 -> overflow_detector/5(s4), s4/1
  sample5_ds/1 -> overflow_detector/6(s5), s5/1
  sample6_ds/1 -> overflow_detector/7(s6), s6/1
  sample7_ds/1 -> overflow_detector/8(s7), s7/1
  sample8_ds/1 -> overflow_detector/9(s8), s8/1
  sample9_ds/1 -> overflow_detector/10(s9), s9/1
  sample10_ds/1 -> overflow_detector/11(s10), s10/1
  sample11_ds/1 -> overflow_detector/12(s11), s11/1
  sample12_ds/1 -> overflow_detector/13(s12), s12/1
  sample13_ds/1 -> overflow_detector/14(s13), s13/1
  sample14_ds/1 -> overflow_detector/15(s14), s14/1
  sample15_ds/1 -> overflow_detector/16(s15), s15/1

== system fft_wideband_real/fft_wideband_real/fft_biplex_real_4x1 ==
  sync : Inport
  shift : Inport  Port=2
  pol1 : Inport  Port=3
  pol2 : Inport  Port=4
  pol3 : Inport  Port=5
  pol4 : Inport  Port=6
  bi_real_unscr_4x : Subsystem
  biplex_core : Subsystem
      settings: AttributesFormatString=|
      | 6 stages
      | reduce logic
      | Virtex5
  ri_to_c_pol1 : Subsystem
  ri_to_c_pol2 : Subsystem
  sync_out : Outport
  pol1_out : Outport  Port=2
  pol2_out : Outport  Port=3
  pol3_out : Outport  Port=4
  pol4_out : Outport  Port=5
  of : Outport  Port=6
  wires:
  pol1/1 -> ri_to_c_pol1/1(re)
  pol2/1 -> ri_to_c_pol1/2(im)
  pol3/1 -> ri_to_c_pol2/1(re)
  pol4/1 -> ri_to_c_pol2/2(im)
  sync/1 -> biplex_core/1(sync)
  shift/1 -> biplex_core/2(shift)
  ri_to_c_pol1/1(c) -> biplex_core/3(pol1)
  ri_to_c_pol2/1(c) -> biplex_core/4(pol2)
  biplex_core/4(of) -> of/1
  biplex_core/1(sync_out) -> bi_real_unscr_4x/1(sync)
  biplex_core/2(out1) -> bi_real_unscr_4x/2(even)
  biplex_core/3(out2) -> bi_real_unscr_4x/3(odd)
  bi_real_unscr_4x/1(sync_out) -> sync_out/1
  bi_real_unscr_4x/2(pol1_out) -> pol1_out/1
  bi_real_unscr_4x/3(pol2_out) -> pol2_out/1
  bi_real_unscr_4x/4(pol3_out) -> pol3_out/1
  bi_real_unscr_4x/5(pol4_out) -> pol4_out/1

== system fft_wideband_real/fft_wideband_real/fft_biplex_real_4x2 ==
  sync : Inport
  shift : Inport  Port=2
  pol1 : Inport  Port=3
  pol2 : Inport  Port=4
  pol3 : Inport  Port=5
  pol4 : Inport  Port=6
  bi_real_unscr_4x : Subsystem
  biplex_core : Subsystem
      settings: AttributesFormatString=|
      | 6 stages
      | reduce logic
      | Virtex5
  ri_to_c_pol1 : Subsystem
  ri_to_c_pol2 : Subsystem
  sync_out : Outport
  pol1_out : Outport  Port=2
  pol2_out : Outport  Port=3
  pol3_out : Outport  Port=4
  pol4_out : Outport  Port=5
  of : Outport  Port=6
  wires:
  pol1/1 -> ri_to_c_pol1/1(re)
  pol2/1 -> ri_to_c_pol1/2(im)
  pol3/1 -> ri_to_c_pol2/1(re)
  pol4/1 -> ri_to_c_pol2/2(im)
  sync/1 -> biplex_core/1(sync)
  shift/1 -> biplex_core/2(shift)
  ri_to_c_pol1/1(c) -> biplex_core/3(pol1)
  ri_to_c_pol2/1(c) -> biplex_core/4(pol2)
  biplex_core/4(of) -> of/1
  biplex_core/1(sync_out) -> bi_real_unscr_4x/1(sync)
  biplex_core/2(out1) -> bi_real_unscr_4x/2(even)
  biplex_core/3(out2) -> bi_real_unscr_4x/3(odd)
  bi_real_unscr_4x/1(sync_out) -> sync_out/1
  bi_real_unscr_4x/2(pol1_out) -> pol1_out/1
  bi_real_unscr_4x/3(pol2_out) -> pol2_out/1
  bi_real_unscr_4x/4(pol3_out) -> pol3_out/1
  bi_real_unscr_4x/5(pol4_out) -> pol4_out/1

== system fft_wideband_real/fft_wideband_real/fft_biplex_real_4x3 ==
  sync : Inport
  shift : Inport  Port=2
  pol1 : Inport  Port=3
  pol2 : Inport  Port=4
  pol3 : Inport  Port=5
  pol4 : Inport  Port=6
  bi_real_unscr_4x : Subsystem
  biplex_core : Subsystem
      settings: AttributesFormatString=|
      | 6 stages
      | reduce logic
      | Virtex5
  ri_to_c_pol1 : Subsystem
  ri_to_c_pol2 : Subsystem
  sync_out : Outport
  pol1_out : Outport  Port=2
  pol2_out : Outport  Port=3
  pol3_out : Outport  Port=4
  pol4_out : Outport  Port=5
  of : Outport  Port=6
  wires:
  pol1/1 -> ri_to_c_pol1/1(re)
  pol2/1 -> ri_to_c_pol1/2(im)
  pol3/1 -> ri_to_c_pol2/1(re)
  pol4/1 -> ri_to_c_pol2/2(im)
  sync/1 -> biplex_core/1(sync)
  shift/1 -> biplex_core/2(shift)
  ri_to_c_pol1/1(c) -> biplex_core/3(pol1)
  ri_to_c_pol2/1(c) -> biplex_core/4(pol2)
  biplex_core/4(of) -> of/1
  biplex_core/1(sync_out) -> bi_real_unscr_4x/1(sync)
  biplex_core/2(out1) -> bi_real_unscr_4x/2(even)
  biplex_core/3(out2) -> bi_real_unscr_4x/3(odd)
  bi_real_unscr_4x/1(sync_out) -> sync_out/1
  bi_real_unscr_4x/2(pol1_out) -> pol1_out/1
  bi_real_unscr_4x/3(pol2_out) -> pol2_out/1
  bi_real_unscr_4x/4(pol3_out) -> pol3_out/1
  bi_real_unscr_4x/5(pol4_out) -> pol4_out/1

== system fft_wideband_real/fft_wideband_real/fft_biplex_real_4x4 ==
  sync : Inport
  shift : Inport  Port=2
  pol1 : Inport  Port=3
  pol2 : Inport  Port=4
  pol3 : Inport  Port=5
  pol4 : Inport  Port=6
  bi_real_unscr_4x : Subsystem
  biplex_core : Subsystem
      settings: AttributesFormatString=|
      | 6 stages
      | reduce logic
      | Virtex5
  ri_to_c_pol1 : Subsystem
  ri_to_c_pol2 : Subsystem
  sync_out : Outport
  pol1_out : Outport  Port=2
  pol2_out : Outport  Port=3
  pol3_out : Outport  Port=4
  pol4_out : Outport  Port=5
  of : Outport  Port=6
  wires:
  bi_real_unscr_4x/5(pol4_out) -> pol4_out/1
  bi_real_unscr_4x/4(pol3_out) -> pol3_out/1
  bi_real_unscr_4x/3(pol2_out) -> pol2_out/1
  bi_real_unscr_4x/2(pol1_out) -> pol1_out/1
  bi_real_unscr_4x/1(sync_out) -> sync_out/1
  biplex_core/3(out2) -> bi_real_unscr_4x/3(odd)
  biplex_core/2(out1) -> bi_real_unscr_4x/2(even)
  biplex_core/1(sync_out) -> bi_real_unscr_4x/1(sync)
  biplex_core/4(of) -> of/1
  ri_to_c_pol2/1(c) -> biplex_core/4(pol2)
  ri_to_c_pol1/1(c) -> biplex_core/3(pol1)
  shift/1 -> biplex_core/2(shift)
  sync/1 -> biplex_core/1(sync)
  pol4/1 -> ri_to_c_pol2/2(im)
  pol3/1 -> ri_to_c_pol2/1(re)
  pol2/1 -> ri_to_c_pol1/2(im)
  pol1/1 -> ri_to_c_pol1/1(re)
